simulink model "untitled2"  (R2014a)
settings: Solver=ode1  SolverMode=SingleTasking  StartTime=0.0  StopTime=T_t  FixedStep=h  RelTol=1e-3
values from neighbouring files (symbols this model uses):
  Ampli_psi2phi = 4    [Parameter.m]
  c1 = 1*beta    (= 0.00349065850399)    [Parameter.m]
  c2 = 400    [Parameter.m]
  Filter_f = 1    [Parameter.m]
  Filter_yes_no = 0    [Parameter.m]
  gainf = 0.3    [Parameter.m]
  h = 0.1    [Parameter.m]
  k1 = 1*0.5*180*beta    (= 0.314159265359)    [Parameter.m]
  m_delay = 0    [Parameter.m]
  mmm = 0.1    [Parameter.m]
  n_mean = 0    [Parameter.m]
  n_var = 0.5    [Parameter.m]
  omega_0 = 0.22    [Parameter.m]
  Tao = 10    [Parameter.m]
  U0 = 7.7175    [Parameter.m]    (also in container.m = 0)
  xi_0 = 0.075    [Parameter.m]
undefined symbols (not defined in the file or in its folder): K_w
settings Model: Creator=Administrator  LastModifiedBy=dittoyi
settings OptimizationCC: ExpressionDepthLimit=2147483647
settings DebuggingCC: UnderspecifiedInitializationDetection=Classic  StateNameClashWarn=warning

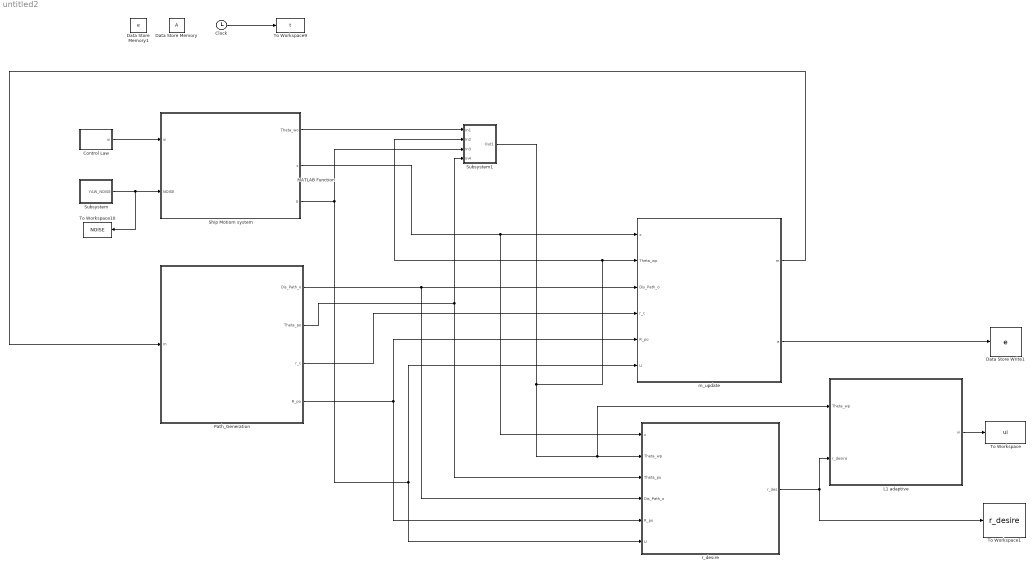
== system untitled2 ==
  Clock : Clock
  Control Law : Subsystem
  Data Store Memory : DataStoreMemory
  Data Store Memory1 : DataStoreMemory  DataStoreName=e
  Data Store Write1 : DataStoreWrite  DataStoreName=e  DataStoreElements=e
  "L1 adaptive " : Subsystem
  MATLAB Function : MATLAB Function  TreatAsAtomicUnit=on
  Path_Generation : Subsystem
  Ship Motiom system : Subsystem
  Subsystem : Subsystem
  Subsystem1 : Subsystem
  To Workspace : ToWorkspace  VariableName=ui  SampleTime=-1
  To Workspace1 : ToWorkspace  VariableName=r_desire  SampleTime=-1
  To Workspace10 : ToWorkspace  VariableName=NOISE  SampleTime=-1
  To Workspace9 : ToWorkspace  VariableName=t  SampleTime=-1
  m_update : Subsystem
  r_desire : Subsystem
  wires:
  Clock/1 -> To Workspace9/1
  Ship Motiom system/2(x) -> r_desire/1(x), m_update/1(x)
  Control Law/1(ui) -> Ship Motiom system/1(ui)
  Path_Generation/2(Theta_po) -> Subsystem1/4(In4), r_desire/3(Theta_po)
  Path_Generation/1(Dis_Path_o) -> r_desire/4(Dis_Path_o), m_update/3(Dis_Path_o)
  Path_Generation/4(R_po) -> r_desire/5(R_po), m_update/5(R_po)
  Path_Generation/3(r_c) -> m_update/4(r_c)
  m_update/1(m) -> Path_Generation/1(m)
  r_desire/1(r_des) -> To Workspace1/1, "L1 adaptive "/2(r_desire)
  Ship Motiom system/3(U) -> r_desire/6(U), m_update/6(U), Subsystem1/3(In3)
  m_update/2(e) -> Data Store Write1/1
  Subsystem/1(YAW_NOISE) -> Ship Motiom system/2(NOISE), To Workspace10/1
  "L1 adaptive "/1(ui) -> To Workspace/1
  Subsystem1/1(Out1) -> "L1 adaptive "/1(Theta_wp), r_desire/2(Theta_wp), Subsystem1/2(In2), m_update/2(Theta_wp)
  Ship Motiom system/1(Theta_wo) -> Subsystem1/1(In1)

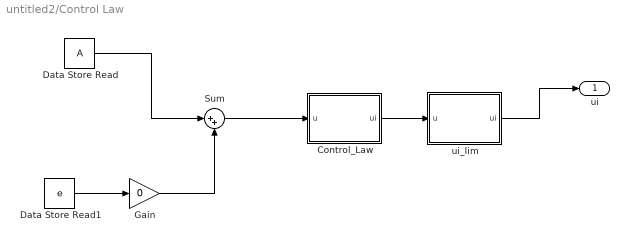
== system untitled2/Control Law ==
  Control_Law : MATLAB Function  TreatAsAtomicUnit=on
  Data Store Read : DataStoreRead  DataStoreElements=A
  Data Store Read1 : DataStoreRead  DataStoreName=e  DataStoreElements=e
  Gain : Gain  Gain=0
  Sum : Sum  Inputs=|++
  ui_lim : MATLAB Function  TreatAsAtomicUnit=on
  ui : Outport
  wires:
  Control_Law/1(ui) -> ui_lim/1(u)
  ui_lim/1(ui) -> ui/1
  Data Store Read1/1 -> Gain/1
  Gain/1 -> Sum/2
  Sum/1 -> Control_Law/1(u)
  Data Store Read/1 -> Sum/1

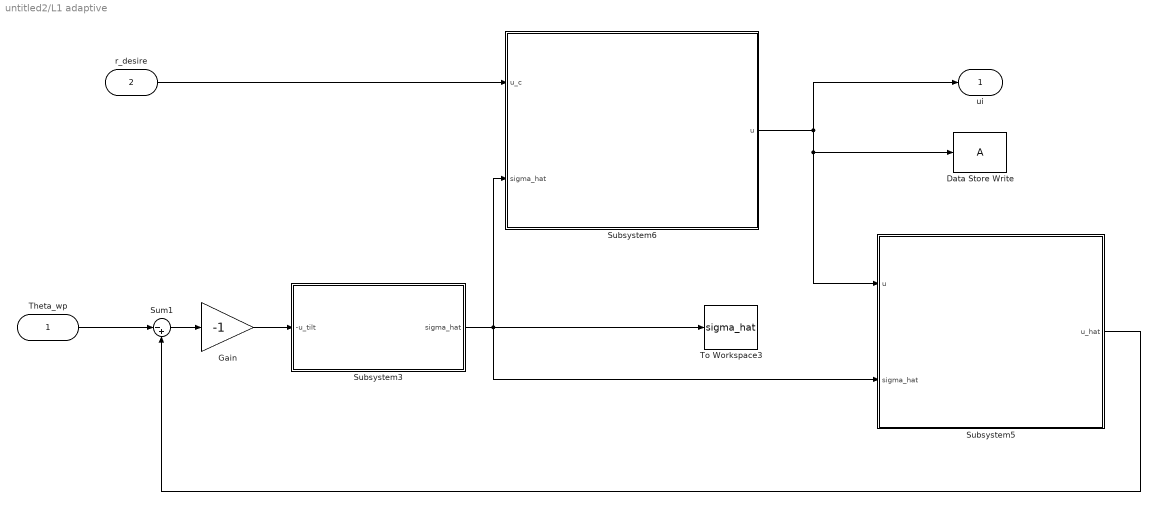
== system untitled2/L1 adaptive  ==
  Theta_wp : Inport
  r_desire : Inport  Port=2
  Data Store Write : DataStoreWrite  DialogController=Simulink.DDGSource
  Gain : Gain  Gain=-1
  Subsystem3 : Subsystem
  Subsystem5 : Subsystem
  Subsystem6 : Subsystem
  Sum1 : Sum  Inputs=|-+
  To Workspace3 : ToWorkspace  VariableName=sigma_hat  SampleTime=-1
  ui : Outport
  wires:
  Subsystem3/1(sigma_hat) -> Subsystem6/2(sigma_hat), To Workspace3/1, Subsystem5/2(sigma_hat)
  Subsystem5/1(u_hat) -> Sum1/2
  Gain/1 -> Subsystem3/1(-u_tilt)
  Sum1/1 -> Gain/1
  Subsystem6/1(u) -> Subsystem5/1(u), Data Store Write/1, ui/1
  Theta_wp/1 -> Sum1/1
  r_desire/1 -> Subsystem6/1(u_c)

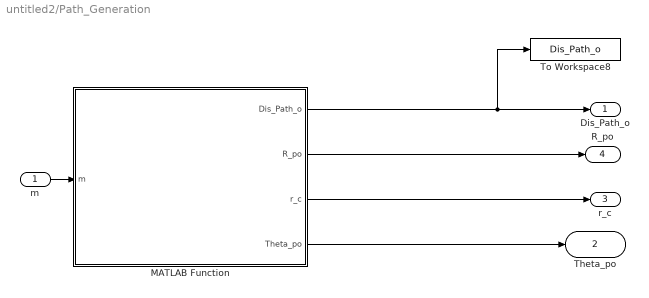
== system untitled2/Path_Generation ==
  m : Inport
  MATLAB Function : MATLAB Function  TreatAsAtomicUnit=on
  To Workspace8 : ToWorkspace  VariableName=Dis_Path_o  SampleTime=-1
  Dis_Path_o : Outport
  Theta_po : Outport  Port=2
  r_c : Outport  Port=3
  R_po : Outport  Port=4
  wires:
  MATLAB Function/2(R_po) -> R_po/1
  m/1 -> MATLAB Function/1(m)
  MATLAB Function/1(Dis_Path_o) -> To Workspace8/1, Dis_Path_o/1
  MATLAB Function/4(Theta_po) -> Theta_po/1
  MATLAB Function/3(r_c) -> r_c/1

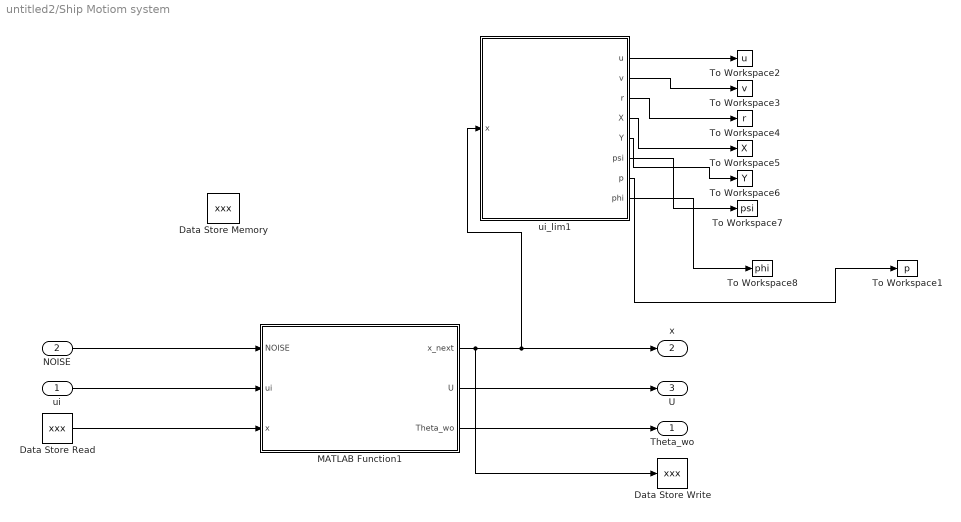
== system untitled2/Ship Motiom system ==
  ui : Inport
  NOISE : Inport  Port=2
  Data Store Memory : DataStoreMemory  DataStoreName=xxx  InitialValue=x_0
  Data Store Read : DataStoreRead  DataStoreName=xxx  DataStoreElements=xxx
  Data Store Write : DataStoreWrite  DataStoreName=xxx  DataStoreElements=xxx
  MATLAB Function1 : MATLAB Function  TreatAsAtomicUnit=on
  To Workspace1 : ToWorkspace  VariableName=p  SampleTime=-1
  To Workspace2 : ToWorkspace  VariableName=u  SampleTime=-1
  To Workspace3 : ToWorkspace  VariableName=v  SampleTime=-1
  To Workspace4 : ToWorkspace  VariableName=r  SampleTime=-1
  To Workspace5 : ToWorkspace  VariableName=X  SampleTime=-1
  To Workspace6 : ToWorkspace  VariableName=Y  SampleTime=-1
  To Workspace7 : ToWorkspace  VariableName=psi  SampleTime=-1
  To Workspace8 : ToWorkspace  VariableName=phi  SampleTime=-1
  ui_lim1 : MATLAB Function  TreatAsAtomicUnit=on
  Theta_wo : Outport
  x : Outport  Port=2
  U : Outport  Port=3
  wires:
  ui_lim1/3(r) -> To Workspace4/1
  MATLAB Function1/2(U) -> U/1
  MATLAB Function1/1(x_next) -> Data Store Write/1, ui_lim1/1(x), x/1
  MATLAB Function1/3(Theta_wo) -> Theta_wo/1
  ui_lim1/1(u) -> To Workspace2/1
  ui_lim1/2(v) -> To Workspace3/1
  ui_lim1/6(psi) -> To Workspace7/1
  ui_lim1/5(Y) -> To Workspace6/1
  ui_lim1/4(X) -> To Workspace5/1
  ui/1 -> MATLAB Function1/2(ui)
  Data Store Read/1 -> MATLAB Function1/3(x)
  NOISE/1 -> MATLAB Function1/1(NOISE)
  ui_lim1/7(p) -> To Workspace1/1
  ui_lim1/8(phi) -> To Workspace8/1

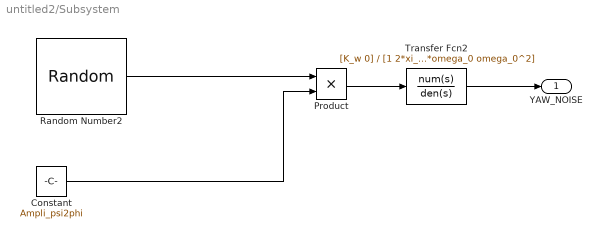
== system untitled2/Subsystem ==
  Constant : Constant  Value=Ampli_psi2phi
  Product : Product  RndMeth=Zero
  Random Number2 : RandomNumber  Mean=n_mean  Variance=n_var  SampleTime=0.1
  Transfer Fcn2 : TransferFcn  Numerator=[K_w 0]  Denominator=[1 2*xi_0*omega_0 omega_0^2]
  YAW_NOISE : Outport
  wires:
  Random Number2/1 -> Product/1
  Constant/1 -> Product/2
  Product/1 -> Transfer Fcn2/1
  Transfer Fcn2/1 -> YAW_NOISE/1

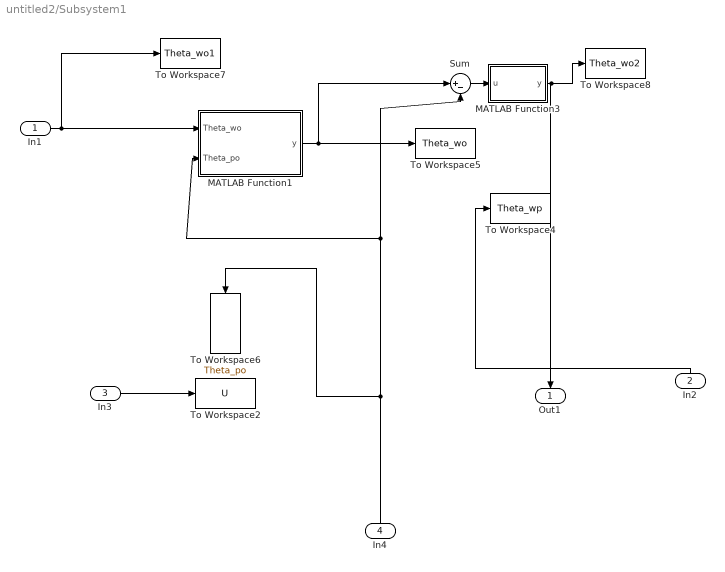
== system untitled2/Subsystem1 ==
  In1 : Inport
  In2 : Inport  Port=2
  In3 : Inport  Port=3
  In4 : Inport  Port=4
  MATLAB Function1 : MATLAB Function  TreatAsAtomicUnit=on
  MATLAB Function3 : MATLAB Function  TreatAsAtomicUnit=on
  Sum : Sum  Inputs=|+-
  To Workspace2 : ToWorkspace  VariableName=U  SampleTime=-1
  To Workspace4 : ToWorkspace  VariableName=Theta_wp  SampleTime=-1
  To Workspace5 : ToWorkspace  VariableName=Theta_wo  SampleTime=-1
  To Workspace6 : ToWorkspace  VariableName=Theta_po  SampleTime=-1
  To Workspace7 : ToWorkspace  VariableName=Theta_wo1  SampleTime=-1
  To Workspace8 : ToWorkspace  VariableName=Theta_wo2  SampleTime=-1
  Out1 : Outport
  wires:
  In1/1 -> To Workspace7/1, MATLAB Function1/1(Theta_wo)
  Sum/1 -> MATLAB Function3/1(u)
  MATLAB Function1/1(y) -> Sum/1, To Workspace5/1
  MATLAB Function3/1(y) -> Out1/1, To Workspace8/1
  In3/1 -> To Workspace2/1
  In2/1 -> To Workspace4/1
  In4/1 -> To Workspace6/1, MATLAB Function1/2(Theta_po), Sum/2

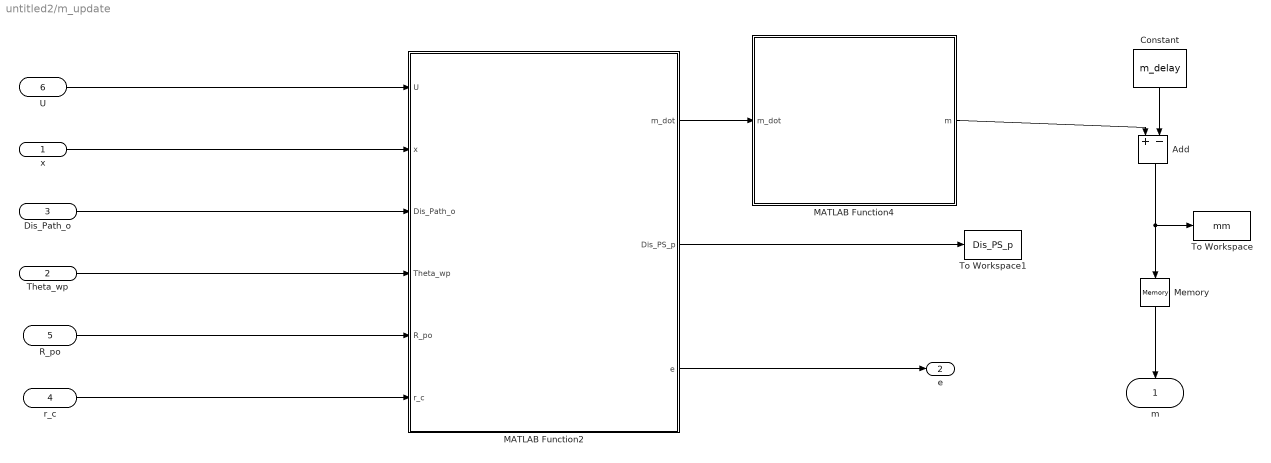
== system untitled2/m_update ==
  x : Inport
  Theta_wp : Inport  Port=2
  Dis_Path_o : Inport  Port=3
  r_c : Inport  Port=4
  R_po : Inport  Port=5
  U : Inport  Port=6
  Add : Sum  Inputs=+-
  Constant : Constant  Value=m_delay
  MATLAB Function2 : MATLAB Function  TreatAsAtomicUnit=on
  MATLAB Function4 : MATLAB Function  TreatAsAtomicUnit=on
  Memory : Memory  X0=[0]  InheritSampleTime=on
  To Workspace : ToWorkspace  VariableName=mm  SampleTime=-1
  To Workspace1 : ToWorkspace  VariableName=Dis_PS_p  SampleTime=-1
  m : Outport
  e : Outport  Port=2
  wires:
  MATLAB Function2/1(m_dot) -> MATLAB Function4/1(m_dot)
  U/1 -> MATLAB Function2/1(U)
  R_po/1 -> MATLAB Function2/5(R_po)
  Dis_Path_o/1 -> MATLAB Function2/3(Dis_Path_o)
  x/1 -> MATLAB Function2/2(x)
  Theta_wp/1 -> MATLAB Function2/4(Theta_wp)
  r_c/1 -> MATLAB Function2/6(r_c)
  Memory/1 -> m/1
  MATLAB Function2/2(Dis_PS_p) -> To Workspace1/1
  MATLAB Function2/3(e) -> e/1
  Constant/1 -> Add/2
  MATLAB Function4/1(m) -> Add/1
  Add/1 -> Memory/1, To Workspace/1

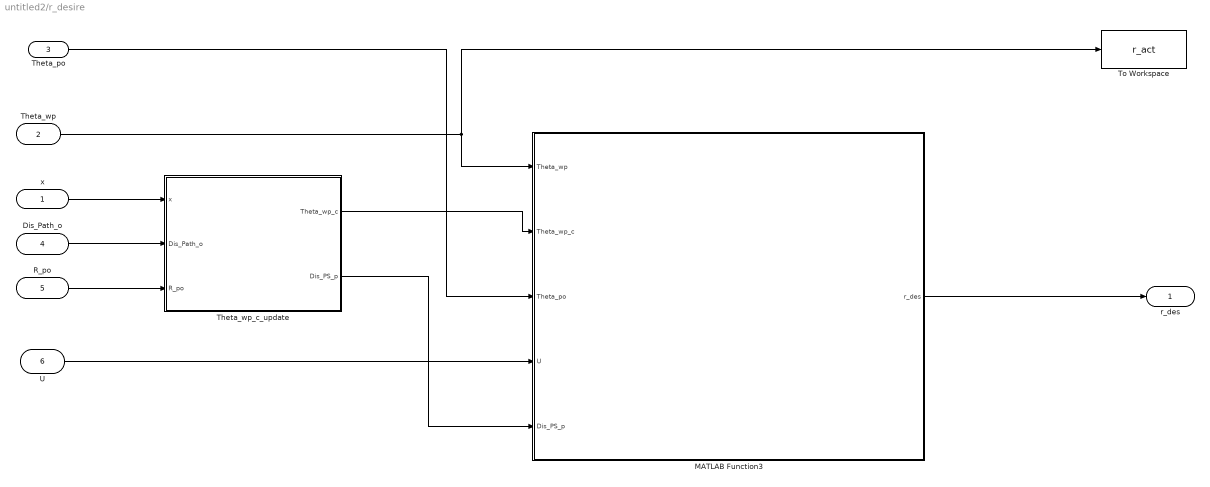
== system untitled2/r_desire ==
  x : Inport
  Theta_wp : Inport  Port=2
  Theta_po : Inport  Port=3
  Dis_Path_o : Inport  Port=4
  R_po : Inport  Port=5
  U : Inport  Port=6
  MATLAB Function3 : MATLAB Function  TreatAsAtomicUnit=on
  Theta_wp_c_update : MATLAB Function  TreatAsAtomicUnit=on
  To Workspace : ToWorkspace  VariableName=r_act  SampleTime=-1
  r_des : Outport
  wires:
  Theta_wp_c_update/1(Theta_wp_c) -> MATLAB Function3/2(Theta_wp_c)
  Theta_wp_c_update/2(Dis_PS_p) -> MATLAB Function3/5(Dis_PS_p)
  Dis_Path_o/1 -> Theta_wp_c_update/2(Dis_Path_o)
  Theta_wp/1 -> MATLAB Function3/1(Theta_wp), To Workspace/1
  R_po/1 -> Theta_wp_c_update/3(R_po)
  x/1 -> Theta_wp_c_update/1(x)
  U/1 -> MATLAB Function3/4(U)
  Theta_po/1 -> MATLAB Function3/3(Theta_po)
  MATLAB Function3/1(r_des) -> r_des/1

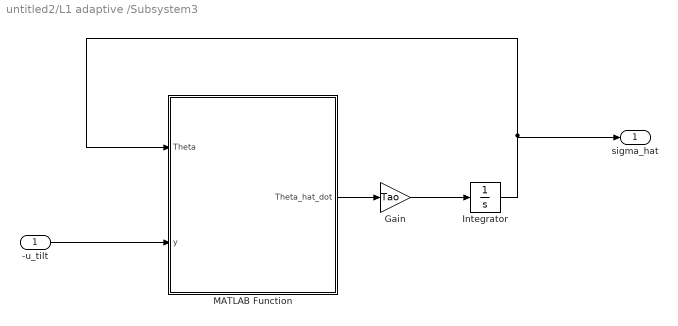
== system untitled2/L1 adaptive /Subsystem3 ==
  -u_tilt : Inport
  Gain : Gain  Gain=Tao
  Integrator : Integrator
  MATLAB Function : MATLAB Function  TreatAsAtomicUnit=on
  sigma_hat : Outport
  wires:
  Integrator/1 -> sigma_hat/1, MATLAB Function/1(Theta)
  -u_tilt/1 -> MATLAB Function/2(y)
  Gain/1 -> Integrator/1
  MATLAB Function/1(Theta_hat_dot) -> Gain/1

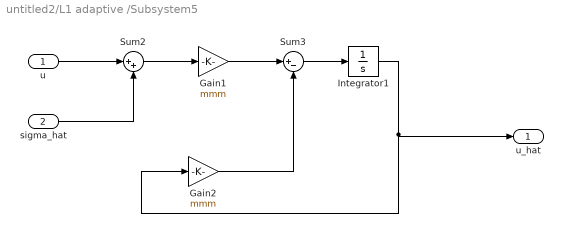
== system untitled2/L1 adaptive /Subsystem5 ==
  u : Inport
  sigma_hat : Inport  Port=2
  Gain1 : Gain  Gain=mmm
  Gain2 : Gain  Gain=mmm
  Integrator1 : Integrator
  Sum2 : Sum  Inputs=|++
  Sum3 : Sum  Inputs=|+-
  u_hat : Outport
  wires:
  sigma_hat/1 -> Sum2/2
  Sum2/1 -> Gain1/1
  Gain2/1 -> Sum3/2
  Integrator1/1 -> u_hat/1, Gain2/1
  u/1 -> Sum2/1
  Sum3/1 -> Integrator1/1
  Gain1/1 -> Sum3/1

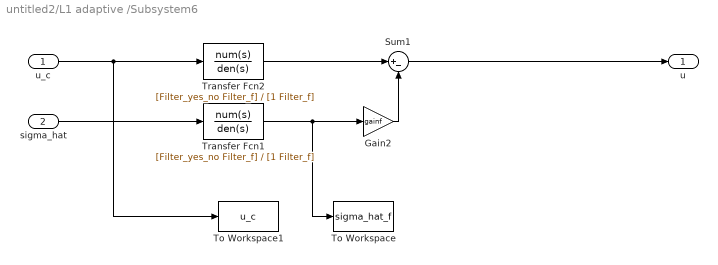
== system untitled2/L1 adaptive /Subsystem6 ==
  u_c : Inport
  sigma_hat : Inport  Port=2
  Gain2 : Gain  Gain=gainf
  Sum1 : Sum  Inputs=|+-
  To Workspace : ToWorkspace  VariableName=sigma_hat_f  SampleTime=-1
  To Workspace1 : ToWorkspace  VariableName=u_c  SampleTime=-1
  Transfer Fcn1 : TransferFcn  Numerator=[Filter_yes_no Filter_f]  Denominator=[1 Filter_f]
  Transfer Fcn2 : TransferFcn  Numerator=[Filter_yes_no Filter_f]  Denominator=[1 Filter_f]
  u : Outport
  wires:
  Gain2/1 -> Sum1/2
  sigma_hat/1 -> Transfer Fcn1/1
  Transfer Fcn1/1 -> Gain2/1, To Workspace/1
  u_c/1 -> Transfer Fcn2/1, To Workspace1/1
  Sum1/1 -> u/1
  Transfer Fcn2/1 -> Sum1/1

== matlab function untitled2/Control Law/ui_lim ==
  data: u input; ui output; h parameter
function ui=ui_lim(u,h)
%global h
persistent u_last;
if isempty(u_last)
    u_last=0;
end

% Parameters, hydrodynamic derivatives and main dimensions
delta_max  = 40;           % max rudder angle      (deg)
Ddelta_max = 5;            % max rudder derivative (deg/s)

ui=u;
if abs(ui) >= delta_max*pi/180,
   ui = sign(u)*delta_max*pi/180;
end
delta_dot = (ui- u_last)/h;

if abs(delta_dot) >= Ddelta_max*pi/180,
   ui = h*sign(delta_dot)*Ddelta_max*pi/180+u_last;
end
u_last=ui;

== matlab function untitled2/Control Law/Control_Law ==
  data: u input; ui output
function ui = fcn(u)
%#codegen

ui = u;

== matlab function untitled2/r_desire/Theta_wp_c_update ==
  data: x input; Dis_Path_o input; Theta_wp_c output; R_po input; Dis_PS_p output; Delta_e parameter
function [Theta_wp_c,Dis_PS_p]=Theta_wp_c_update(x,Dis_Path_o,R_po,Delta_e)
%global Delta_e
 Dis_Ship_o=[x(4) x(5)]';
%[Dis_Path_o,R_po,r_c,Theta_po]=Path_Generation(m);
Dis_PS_p=R_po*(Dis_Ship_o-Dis_Path_o)
Theta_wp_c=atan(-Dis_PS_p(2)/(Delta_e));

== matlab function untitled2/Path_Generation/MATLAB Function ==
  data: m input; Dis_Path_o output; R_po output; r_c output; Theta_po output
function [Dis_Path_o,R_po,r_c,Theta_po]=Path_Generation(m) %[Dis_Path_o,R_po,r_c,Theta_po]=Path_Generation(m)
%m=m(length(m));
%y=m;
%
ww=0.3;
x=1500*sin(0.01*m);
y=1500*cos(0.01*m);
x_dot=15*cos(0.01*m);
y_dot=-15*sin(0.01*m);

% 
% x=200*m;
% y=100*m;
% x_dot=200;
% y_dot=100;


Dis_Path_o=[x,y]';
R_po=[x_dot/(sqrt(x_dot^2+y_dot^2)) y_dot/(sqrt(x_dot^2+y_dot^2));-y_dot/(sqrt(x_dot^2+y_dot^2)) x_dot/(sqrt(x_dot^2+y_dot^2))];
r_c=sqrt(x_dot^2+y_dot^2);

Theta_po=(1+sign(abs(y_dot)))/2*(1-sign(x_dot))*sign(y_dot)*pi/2+atan(y_dot/x_dot);

% 
% if x_dot=0
%     if y_dot<0
%         Theta_po=-pi/2;
%     else if y_dot>0
%             Theta_po=pi/2;
%         end
%     end
% end
% 
% if x_dot<0
%     if y_dot<0
%         Theta_po=-pi/2+atan(y_dot/x_dot);
%     else if y_dot>0
%             Theta_po=pi/2+atan(y_dot/x_dot);
%         end
%     end
% end
%

== matlab function untitled2/Ship Motiom system/MATLAB Function1 ==
  data: NOISE input; x_next output; ui input; U output; Theta_wo output; U0 parameter; h parameter; x input
function [x_next,U,Theta_wo]=Fourth_Order_Runge_Kutta(NOISE,ui,U0,h,x)
%
% u     = pertubed surge velocity about Uo (m/s)
% v     = pertubed sway velocity about zero (m/s)
% r     = pertubed yaw velocity about zero (rad/s)
% x     = position in x-direction (m)
% y     = position in y-direction (m)
% psi   = pertubed yaw angle about zero (rad)
% delta = actual rudder angle (rad)
%
% The inputs are :
% 
% ui    = commanded rudder angle (rad)
% U0    = nominal speed (optionally). Default value is U0 = 7.7175 m/s = 15 knots.
%
%global U0 h x_0;

[k1,U1]=container(x,ui,U0,NOISE);
[k2,U2]=container(x+h/2*k1,ui,U0,NOISE);
[k3,U3]=container(x+h/2*k2,ui,U0,NOISE);
[k4,U4]=container(x+h*k3,ui,U0,NOISE);
x_next=x+h*(k1+2*k2+2*k3+k4)/6;
ddd=(k1+2*k2+2*k3+k4)/6
U=(U1+2*U2+2*U3+U4)/6;
Theta_bo=x_next(6);
Theta_wb=atan(x_next(2)/U);
Theta_wo=atan(x_next(2)/U)+Theta_bo;
%x=x_next;

== matlab function untitled2/m_update/MATLAB Function2 ==
  data: U input; m_dot output; x input; Dis_Path_o input; Theta_wp input; R_po input; r_c input; gama parameter; Dis_PS_p output; e output
function [m_dot, Dis_PS_p,e]=m_update(U,x,Dis_Path_o,Theta_wp,R_po,r_c,gama)
%global gama;
Dis_Ship_o=[x(4) x(5)]';
%[Dis_Path_o,R_po,r_c,Theta_po]=Path_Generation(m);
Dis_PS_p=R_po*(Dis_Ship_o-Dis_Path_o);
e=Dis_PS_p(2);
m_dot=(U*cos(Theta_wp)+gama*Dis_PS_p(1))/r_c;

== matlab function untitled2/r_desire/MATLAB Function3 ==
  data: Theta_wp input; r_des output; Theta_wp_c input; Theta_po input; U input; Dis_PS_p input; c1 parameter; c2 parameter; k1 parameter; h parameter
function r_des =r_desire(Theta_wp,Theta_wp_c,Theta_po,U,Dis_PS_p,c1, c2, k1, h)
%global c1 c2 c3 h;
persistent Theta_wp_c_last;
if isempty(Theta_wp_c_last)
    Theta_wp_c_last=0;
end
Theta_wp_c_dot=0*(Theta_wp_c-Theta_wp_c_last)/h;

persistent Theta_po_last;
if isempty(Theta_po_last)
    Theta_po_last=0;
end

%Theta_po_dot=(Theta_po-Theta_po_last)/h
if abs(Theta_wp-Theta_wp_c)<0.01
    r_des=Theta_wp_c_dot-k1*(Theta_wp-Theta_wp_c)-c1*U*Dis_PS_p(2)/c2;
else
r_des=Theta_wp_c_dot-k1*(Theta_wp-Theta_wp_c)-c1*U*Dis_PS_p(2)*(sin(Theta_wp)-sin(Theta_wp_c))/(c2*(Theta_wp-Theta_wp_c));
end

%r_des=r_des1(1);
Theta_po_last=Theta_po;
Theta_wp_c_last=Theta_wp_c;

== matlab function untitled2/m_update/MATLAB Function4 ==
  data: m_dot input; m output; h parameter
function m = fcn(m_dot,h)
%#codegen
%global h;
persistent m_last;
if isempty(m_last)
    m_last=0;
end
m=m_last+h*m_dot;
m_last=m;

== matlab function untitled2/Ship Motiom system/ui_lim1 ==
  data: u output; v output; x input; r output; X output; Y output; psi output; p output; phi output
function [u,v,r,X,Y,psi,p,phi]=Demux(x)
u=x(1);v=x(2);r=x(3);X=x(4);Y=x(5);psi=x(6);p=x(7);phi=x(8);

== matlab function untitled2/L1 adaptive /Subsystem3/MATLAB Function ==
  data: Theta input; Theta_hat_dot output; y input
function Theta_hat_dot = Proj(Theta,y)
%#codegen
e_theta=0.5;Theta_max=20;
f_theta=((e_theta+1)*Theta'*Theta-Theta_max^2)/(e_theta*Theta_max^2);
Delta_f=2*(e_theta+1)/(e_theta*Theta_max^2)*[Theta]';
%y=x*x_tild'*P*b;
Delta_f_norm=Delta_f/norm(Delta_f);
%y=[nan nan]';
if (f_theta<0)
    Theta_hat_dot=y;
elseif (f_theta>=0 & Delta_f'*y<=0)
    Theta_hat_dot=y;
else (f_theta>=0 & Delta_f'*y>0)
    Theta_hat_dot=y-Delta_f_norm*(Delta_f_norm'*y)*f_theta;
end

== matlab function untitled2/MATLAB Function ==
  data: u input; y output
function y = fcn(u)
%#codegen

y = u;

== matlab function untitled2/Subsystem1/MATLAB Function1 ==
  data: Theta_wo input; y output; Theta_po input
function y = fcn(Theta_wo,Theta_po)
%codegen
we=sign(Theta_wo)*mod(abs(Theta_wo)*180/pi,360)/180*pi;
we2=we-2*pi;%we-1.5*pi*(1+sign(we-pi/2))/2;
y=(1+sign(Theta_po))/2*we+(1-sign(Theta_po))/2*we2;

%y=sign(Theta_wo)*mod(abs(Theta_wo)*180/pi,360)/180*pi-(1-sign(Theta_po))*pi;
%

== matlab function untitled2/Subsystem1/MATLAB Function3 ==
  data: u input; y output
function y = fcn(u)
%#codegen
a1=(1-sign(abs(u)-pi))/2;
a2=(1+sign(abs(u)-pi))/2;
k3=-sign(u)*(2*pi-abs(u));
y=a1*u+a2*k3;
%y=sign(u)*abs((abs(u)-(1+sign(abs(u)-pi))*pi));
%mod(abs(u)/pi*180,90)*pi/180;
%
